simulink model "es2_sim"  (Simulink 7.0)
settings: Solver=ode45  StartTime=0.0  StopTime=10  MaxStep=0.1  RelTol=1e-3  AbsTol=1e-3
values from neighbouring files (symbols this model uses):
  A = [-5 -11;4 7]    [es1a.m]    (also in es2a.m = [11 29;-5 -12])
  B = [1 1]'    [es1a.m]    (also in es2a.m)
  C = [1 0]    [es1a.m]    (also in es2a.m)
  K = place(A,B,autoval)    [es2a.m]
  L = place(A',C',[-40 -50])'    [es2a.m]
settings Model: Creator=claudio  LastModifiedBy=claudio  ExtModeTrigMode=oneshot  ExtModeArmWhenConnect=off
settings DataIOCC: LimitDataPoints=off  SaveOutput=off  SaveTime=off
settings OptimizationCC: BooleanDataType=off  InlineInvariantSignals=on
settings DebuggingCC: SaveWithParameterizedLinksMsg=none  SignalResolutionControl=TryResolveAllWithWarning  SolverPrmCheckMsg=none  MultiTaskDSMMsg=warning  MultiTaskCondExecSysMsg=none  StrictBusMsg=None
settings HardwareCC: TargetUnknown=on
settings RTWCC: IncludeERTFirstTime=on
settings GRTTargetCC: TargetFcnLib=ansi_tfl_tmw.mat  ModelReferenceCompliant=off  MatFileLogging=off

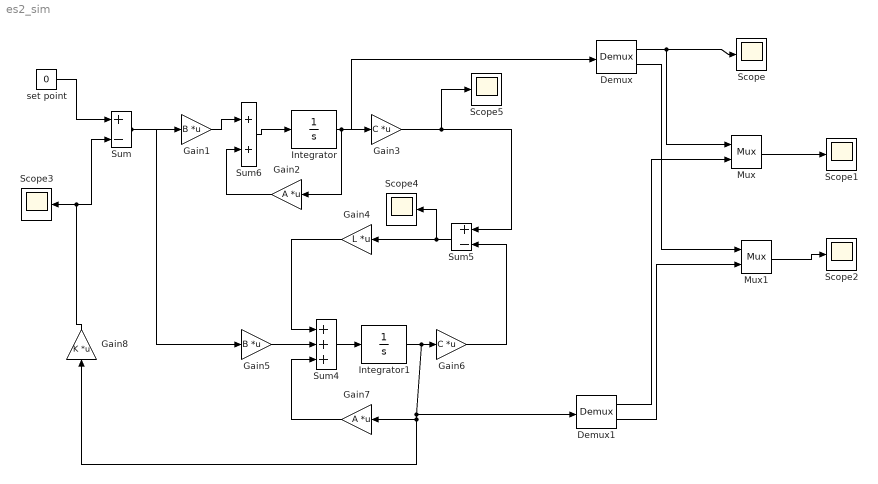
== system es2_sim ==
  Demux : Demux  Outputs=2
  Demux1 : Demux  Outputs=2
  Gain1 : Gain  Gain=B  Multiplication=Matrix(K*u)  ParameterDataType=sfix(16)  ParameterScaling=2^0  OutDataType=sfix(16)  OutScaling=2^0
  Gain2 : Gain  Orientation=left  Gain=A  Multiplication=Matrix(K*u)  ParameterDataType=sfix(16)  ParameterScaling=2^0  OutDataType=sfix(16)  OutScaling=2^0
  Gain3 : Gain  Gain=C  Multiplication=Matrix(K*u)  ParameterDataType=sfix(16)  ParameterScaling=2^0  OutDataType=sfix(16)  OutScaling=2^0
  Gain4 : Gain  Orientation=left  Gain=L  Multiplication=Matrix(K*u)  ParameterDataType=sfix(16)  ParameterScaling=2^0  OutDataType=sfix(16)  OutScaling=2^0
  Gain5 : Gain  Gain=B  Multiplication=Matrix(K*u)  ParameterDataType=sfix(16)  ParameterScaling=2^0  OutDataType=sfix(16)  OutScaling=2^0
  Gain6 : Gain  Gain=C  Multiplication=Matrix(K*u)  ParameterDataType=sfix(16)  ParameterScaling=2^0  OutDataType=sfix(16)  OutScaling=2^0
  Gain7 : Gain  Orientation=left  Gain=A  Multiplication=Matrix(K*u)  ParameterDataType=sfix(16)  ParameterScaling=2^0  OutDataType=sfix(16)  OutScaling=2^0
  Gain8 : Gain  Orientation=up  Gain=K  Multiplication=Matrix(K*u)  ParameterDataType=sfix(16)  ParameterScaling=2^0  OutDataType=sfix(16)  OutScaling=2^0
  Integrator : Integrator  InitialCondition=[3 5]
  Integrator1 : Integrator  InitialCondition=[ 0 0 ]
  Mux : Mux  Inputs=2
  Mux1 : Mux  Inputs=2
  Scope{,1..5} (6 alike) : Scope
      Scope settings: TimeRange=10
      Scope2 settings: SaveName=ScopeData2
      Scope3 settings: SaveName=ScopeData3
      Scope4 settings: SaveName=ScopeData4
      Scope5 settings: TimeRange=10  SaveName=ScopeData5
  Sum : Sum  Inputs=+-  OutDataType=sfix(16)  OutScaling=2^0  SaturateOnIntegerOverflow=on  InputSameDT=on
  Sum4 : Sum  Inputs=+++  OutDataType=sfix(16)  OutScaling=2^0  SaturateOnIntegerOverflow=on  InputSameDT=on
  Sum5 : Sum  Orientation=left  Inputs=+-  OutDataType=sfix(16)  OutScaling=2^0  SaturateOnIntegerOverflow=on  InputSameDT=on
  Sum6 : Sum  OutDataType=sfix(16)  OutScaling=2^0  SaturateOnIntegerOverflow=on  InputSameDT=on
  set point : Constant  Value=0  OutDataType=sfix(16)  OutScaling=2^0
  wires:
  Integrator1/1 -> Demux1/1, Gain7/1, Gain8/1, Gain6/1
  Sum4/1 -> Integrator1/1
  Gain7/1 -> Sum4/3
  Gain5/1 -> Sum4/2
  Gain3/1 -> Scope5/1, Sum5/1
  Gain6/1 -> Sum5/2
  Gain4/1 -> Sum4/1
  Integrator/1 -> Demux/1, Gain2/1, Gain3/1
  Sum5/1 -> Gain4/1, Scope4/1
  Sum6/1 -> Integrator/1
  Gain8/1 -> Sum/2, Scope3/1
  set point/1 -> Sum/1
  Gain2/1 -> Sum6/2
  Sum/1 -> Gain1/1, Gain5/1
  Demux1/1 -> Mux/2
  Demux/1 -> Mux/1, Scope/1
  Mux/1 -> Scope1/1
  Demux/2 -> Mux1/1
  Demux1/2 -> Mux1/2
  Mux1/1 -> Scope2/1
  Gain1/1 -> Sum6/1
